simulink subsystem "MCD"  (R2025a)
settings: Solver=VariableStepAuto  StartTime=0.0  StopTime=10.0  RelTol=1e-3
undefined symbols (not defined in the file): d
settings Model: Creator=Antonio  LastModifiedBy=aj
settings RTWCC: GPUComputeCapability=3.5

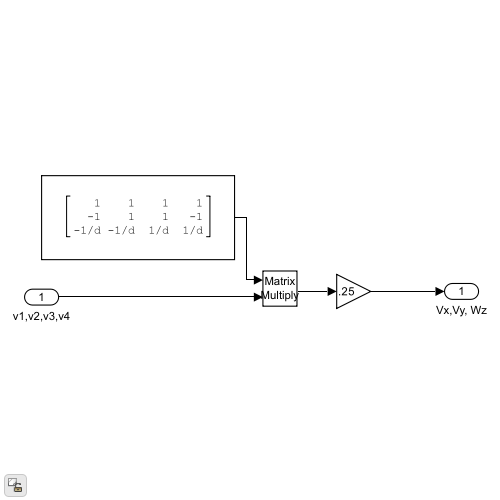
[thumbnail: Simulink's stored preview of the top-level diagram]
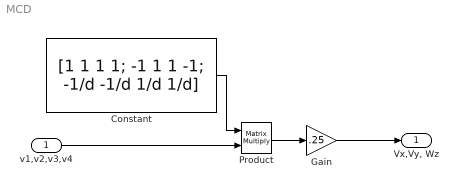
== system MCD ==
  v1,v2,v3,v4 : Inport
  Constant : Constant  Value="[1  1 1 1; -1 1 1 -1;  -1/d -1/d 1/d 1/d]"
  Gain : Gain  Gain=.25
  Product : Product  Multiplication=Matrix(*)
  "Vx,Vy, Wz" : Outport
  wires:
  Constant/1 -> Product/1
  v1,v2,v3,v4/1 -> Product/2
  Product/1 -> Gain/1
  Gain/1 -> "Vx,Vy, Wz"/1
